simulink model "MotorSoftStart_2025a"  (R2025a)
settings: Solver=VariableStepAuto  StartTime=0.0  StopTime=10.0  RelTol=1e-3
libraries: simulink x1
settings Model: Creator=mahij  LastModifiedBy=mahij

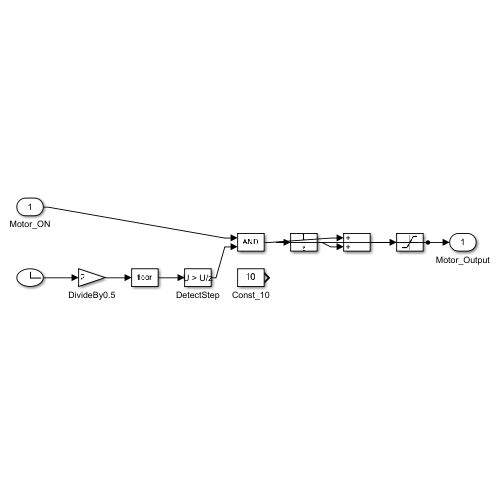
[thumbnail: Simulink's stored preview of the top-level diagram]
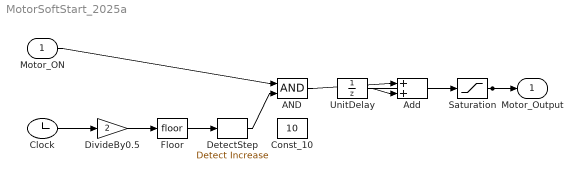
== system MotorSoftStart_2025a ==
  Motor_ON : Inport
  AND : Logic  AllPortsSameDT=off  OutDataTypeStr=boolean
  Add : Sum
  Clock : Clock
  Const_10 : Constant  Value=10
  DetectStep : simulink/Logic and Bit Operations/Detect Increase  vinit=0.0  OutDataTypeStr=boolean
  DivideBy0.5 : Gain  Gain=2
  Floor : Rounding
  Saturation : Saturate  UpperLimit=100  LowerLimit=0
  UnitDelay : UnitDelay  SampleTime=0.5  HasFrameUpgradeWarning=on
  Motor_Output : Outport
  wires:
  Motor_ON/1 -> AND/1
  Clock/1 -> DivideBy0.5/1
  DivideBy0.5/1 -> Floor/1
  Floor/1 -> DetectStep/1
  DetectStep/1 -> AND/2
  AND/1 -> Add/1
  UnitDelay/1 -> Add/2
  Add/1 -> Saturation/1
  Saturation/1 -> Motor_Output/1, UnitDelay/1
